simulink model "twoBodySim_cartesian"  (R2014a)
settings: Solver=ode45  StartTime=0.0  StopTime=Tsim  RelTol=1e-10  AbsTol=1e-10
values from neighbouring files (symbols this model uses):
  fixPositionOfMass1 = 1    [script02_simulate_earths_orbit.m]    (also in script03_simulate_eccentric_orbit.m; script04_twoEqualMassObjects.m = 0; script05_plutoAndCharon.m = 0; script06_threeBodySim.m = 0)
  G = 6.674e-11    [calcTwoBodyPlaneDynamics.m]    (also in script02_simulate_earths_orbit.m; script03_simulate_eccentric_orbit.m; script04_twoEqualMassObjects.m; script05_plutoAndCharon.m)
  m1 = 2e30    (= 2e+30)    [script02_simulate_earths_orbit.m]    (also in script03_simulate_eccentric_orbit.m; script04_twoEqualMassObjects.m = 1e+22; script05_plutoAndCharon.m = 1.3e+22; script06_threeBodySim.m = 1.3e+22)
  m2 = 1    [script02_simulate_earths_orbit.m]    (also in script03_simulate_eccentric_orbit.m; script04_twoEqualMassObjects.m = 1e+22; script05_plutoAndCharon.m = 1.5e+21; script06_threeBodySim.m = 1.5e+21)
  r1_init = -r2_init*1e-6    [script02_simulate_earths_orbit.m]    (also in script03_simulate_eccentric_orbit.m; script04_twoEqualMassObjects.m = -r2_init; script05_plutoAndCharon.m = r1; script06_threeBodySim.m = r1)
  r1dot_init = -r2dot_init*1e-6    [script02_simulate_earths_orbit.m]    (also in script03_simulate_eccentric_orbit.m; script04_twoEqualMassObjects.m = -r2dot_init; script05_plutoAndCharon.m = r1dot; script06_threeBodySim.m = r1dot)
  r2_init = [149e9 0, 0]'    [script02_simulate_earths_orbit.m]    (also in script03_simulate_eccentric_orbit.m; script04_twoEqualMassObjects.m = [1e8 0, 0]'; script05_plutoAndCharon.m = r2; script06_threeBodySim.m = r2)
  r2dot_init = [0, 29.78e3,0]'    [script02_simulate_earths_orbit.m]    (also in script03_simulate_eccentric_orbit.m = [0, 29.78e3*0.5,0]'; script04_twoEqualMassObjects.m = [0, sqrt(G*m1/(4*r2_init(1)))*0.5,0]'; script05_plutoAndCharon.m = r2dot; script06_threeBodySim.m = r2dot)
  scaleFac = 1e6    (= 1000000)    [script02_simulate_earths_orbit.m]    (also in script03_simulate_eccentric_orbit.m; script04_twoEqualMassObjects.m = 1; script05_plutoAndCharon.m = 10^(floor(log10(R_low))); script06_threeBodySim.m = 10^(floor(log10(R_low))))
libraries: simulink x2
settings Model: Creator=Timo  LastModifiedBy=Timo

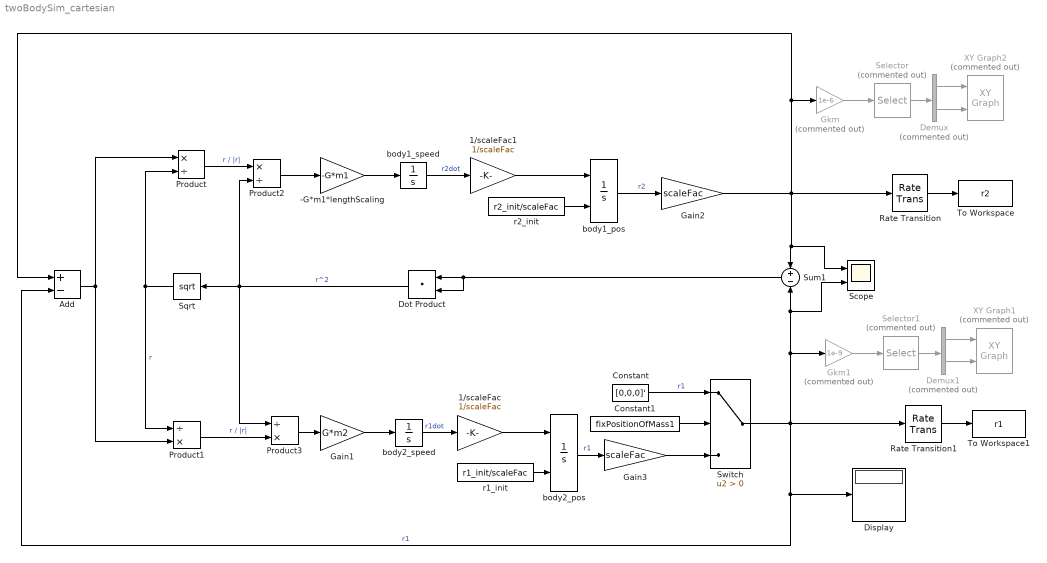
== system twoBodySim_cartesian ==
  -G*m1*lengthScaling : Gain  Gain=-G*m1
  1/scaleFac : Gain  Gain=1/scaleFac
  1/scaleFac1 : Gain  Gain=1/scaleFac
  Add : Sum  Inputs=+-
  Constant : Constant  Value=[0,0,0]'
  Constant1 : Constant  Value=fixPositionOfMass1
  Demux : Demux  Commented=on  Outputs=2
  Demux1 : Demux  Commented=on  Outputs=2
  Display : Display
  Dot Product : DotProduct  InputSameDT=on  OutDataTypeStr=Inherit: Inherit via internal rule
  Gain1 : Gain  Gain=G*m2
  Gain2 : Gain  Gain=scaleFac
  Gain3 : Gain  Gain=scaleFac
  Gkm : Gain  Commented=on  Gain=1e-6
  Gkm1 : Gain  Commented=on  Gain=1e-9
  Product : Product  Inputs=*/
  Product1 : Product  Inputs=/*
  Product2 : Product  Inputs=*/
  Product3 : Product  Inputs=/*
  Rate Transition : RateTransition  OutPortSampleTime=T_sample
  Rate Transition1 : RateTransition  OutPortSampleTime=T_sample
  Scope : Scope  NumInputPorts=2
      settings: YMin=-2e+07~-2.25e+06  YMax=2e+07~2.25e+06
  Selector : Selector  Commented=on  InputPortWidth=3  Indices=[1 2]
  Selector1 : Selector  Commented=on  InputPortWidth=3  Indices=[1 2]
  Sqrt : Sqrt  SaturateOnIntegerOverflow=on
  Sum1 : Sum  Inputs=+-
  Switch : Switch  Criteria=u2 > Threshold
  To Workspace : ToWorkspace  VariableName=r2  SaveFormat=Timeseries  SampleTime=-1
  To Workspace1 : ToWorkspace  VariableName=r1  SaveFormat=Timeseries  SampleTime=-1
  XY Graph1 : simulink/Sinks/XY Graph  Commented=on  xmin=-r2_init(1)*1.5  xmax=r2_init(1)*1.5  ymin=-r2_init(1)*1.5  ymax=r2_init(1)*1.5  st=-1
  XY Graph2 : simulink/Sinks/XY Graph  Commented=on  xmin=-r2_init(1)*1.5  xmax=r2_init(1)*1.5  ymin=-r2_init(1)*1.5  ymax=r2_init(1)*1.5  st=-1
  body1_pos : Integrator  InitialConditionSource=external  InitialCondition=r2_init
  body1_speed : Integrator  InitialCondition=r2dot_init
  body2_pos : Integrator  InitialConditionSource=external  InitialCondition=r1_init
  body2_speed : Integrator  InitialCondition=r1dot_init
  r1_init : Constant  Value=r1_init/scaleFac
  r2_init : Constant  Value=r2_init/scaleFac
  wires:
  body1_speed/1 -> 1/scaleFac1/1  "r2dot"
  body2_speed/1 -> 1/scaleFac/1  "r1dot"
  Switch/1 -> Gkm1/1, Scope/2, Sum1/2, Add/2, Display/1, Rate Transition1/1  "r1"
  Product1/1 -> Product3/2  "r / |r|"
  body1_pos/1 -> Gain2/1  "r2"
  Demux/1 -> XY Graph2/1
  Add/1 -> Product/1, Product1/2
  Sqrt/1 -> Product/2, Product1/1  "r"
  Product2/1 -> -G*m1*lengthScaling/1
  Product/1 -> Product2/1  "r / |r|"
  Selector/1 -> Demux/1
  Gkm/1 -> Selector/1
  body2_pos/1 -> Gain3/1  "r1"
  Constant/1 -> Switch/1  "r1"
  Rate Transition/1 -> To Workspace/1
  Rate Transition1/1 -> To Workspace1/1
  Constant1/1 -> Switch/2
  Demux/2 -> XY Graph2/2
  Selector1/1 -> Demux1/1
  Gkm1/1 -> Selector1/1
  Demux1/2 -> XY Graph1/2
  Demux1/1 -> XY Graph1/1
  Product3/1 -> Gain1/1
  Dot Product/1 -> Product3/1, Sqrt/1, Product2/2  "r^2"
  Sum1/1 -> Dot Product/2, Dot Product/1
  Gain2/1 -> Sum1/1, Scope/1, Gkm/1, Add/1, Rate Transition/1
  Gain3/1 -> Switch/3
  Gain1/1 -> body2_speed/1
  -G*m1*lengthScaling/1 -> body1_speed/1
  1/scaleFac1/1 -> body1_pos/1
  r2_init/1 -> body1_pos/2
  r1_init/1 -> body2_pos/2
  1/scaleFac/1 -> body2_pos/1
